simulink model "cw5_model_Relidzynski"  (R2017b)
settings: Solver=VariableStepAuto  StartTime=0.0  StopTime=30.0  RelTol=1e-3
values from neighbouring files (symbols this model uses):
  A = [0,1;-a0,-a1]    [cw5_dane_Relidzynski.m]
  a0 = h/m    (= 3.2)    [cw5_dane_Relidzynski.m]
  a1 = a/m    (= 0.8)    [cw5_dane_Relidzynski.m]
  B = [0;b0]    [cw5_dane_Relidzynski.m]
  b0 = 1/m    (= 16)    [cw5_dane_Relidzynski.m]
  C = [1,0]    [cw5_dane_Relidzynski.m]
  D = [0]    [cw5_dane_Relidzynski.m]
settings Model: Creator=Radosław  LastModifiedBy=Radosław
settings DataIOCC: ReturnWorkspaceOutputs=on
settings DebuggingCC: UnconnectedInputMsg=none  UnconnectedOutputMsg=none  UnconnectedLineMsg=none  SFMachineParentedDataDiag=error
settings SFSimCC: SimUseLocalCustomCode=on
settings RTWCC: RTWUseLocalCustomCode=on

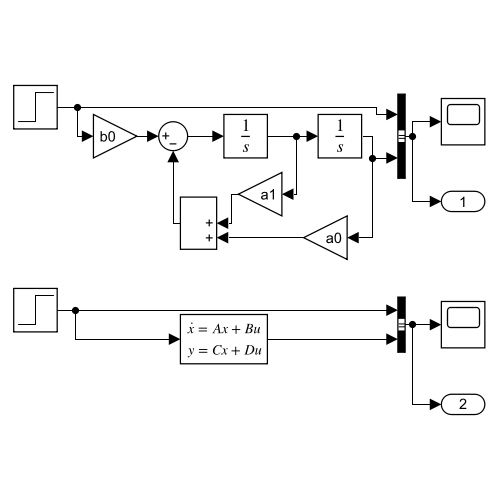
[thumbnail: Simulink's stored preview of the top-level diagram]
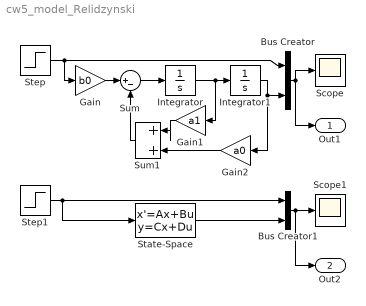
== system cw5_model_Relidzynski ==
  Bus Creator : BusCreator  Inputs=2
  Bus Creator1 : BusCreator  Inputs=2
  Gain : Gain  Gain=b0
  Gain1 : Gain  Gain=a1
  Gain2 : Gain  Gain=a0
  Integrator : Integrator
  Integrator1 : Integrator
  Scope : Scope
  Scope1 : Scope
  State-Space : StateSpace  A=A  B=B  C=C  D=D  InitialCondition=0
  Step : Step  Time=0  SampleTime=0
  Step1 : Step  Time=0  SampleTime=0
  Sum : Sum  Inputs=|+-
  Sum1 : Sum  Inputs=|++
  Out1 : Outport
  Out2 : Outport  Port=2
  wires:
  Step/1 -> Gain/1, Bus Creator/1
  Gain/1 -> Sum/1
  Sum/1 -> Integrator/1
  Integrator/1 -> Gain1/1, Integrator1/1
  Integrator1/1 -> Gain2/1, Bus Creator/2
  Gain1/1 -> Sum1/1
  Gain2/1 -> Sum1/2
  Sum1/1 -> Sum/2
  Bus Creator/1 -> Scope/1, Out1/1
  Bus Creator1/1 -> Out2/1, Scope1/1
  Step1/1 -> State-Space/1, Bus Creator1/1
  State-Space/1 -> Bus Creator1/2
